simulink subsystem "sensor"  (R2023b)
settings: Solver=VariableStepAuto  StartTime=0.0  StopTime=10.0  RelTol=1e-3
libraries: arduinolib x2
settings Model: Creator=Usuario_UMA  LastModifiedBy=Usuario_UMA

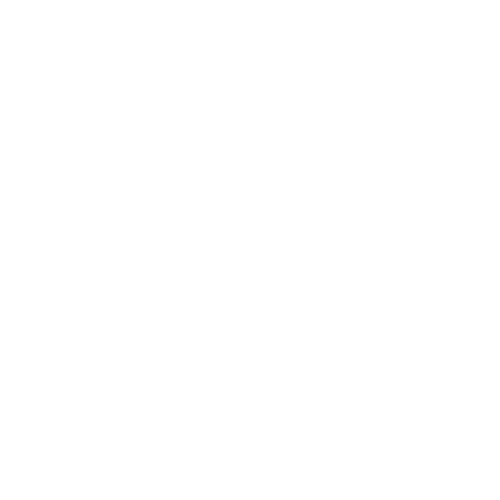
[thumbnail: Simulink's stored preview of the top-level diagram]
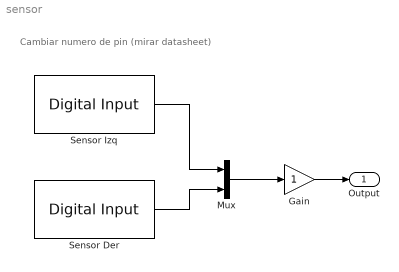
== system sensor ==
  note: Cambiar numero de pin (mirar datasheet)
  Gain : Gain
  Mux : Mux  Inputs=2
  Sensor Der : arduinolib/Digital Input  pinNumber=8  mode=Default  Direction=input  SampleTime=0.1  blockPlatform=arduino
  Sensor Izq : arduinolib/Digital Input  pinNumber=8  mode=Default  Direction=input  SampleTime=0.1  blockPlatform=arduino
  Output : Outport
  wires:
  Sensor Der/1 -> Mux/2
  Sensor Izq/1 -> Mux/1
  Mux/1 -> Gain/1
  Gain/1 -> Output/1
